simulink model "ex5_3_flowchart"  (R2018b)
settings: Solver=VariableStepAuto  StartTime=0.0  StopTime=20  RelTol=1e-3
settings Model: Creator=HYJ  LastModifiedBy=HYJ

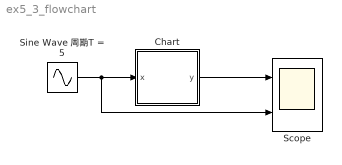
== system ex5_3_flowchart ==
  Chart : Stateflow chart  TreatAsAtomicUnit=on
  Scope : Scope  NumInputPorts=2
  Sine Wave 周期T = 5 : Sin  Frequency=0.2  SampleTime=0
  wires:
  Sine Wave 周期T = 5/1 -> Scope/2, Chart/1(x)
  Chart/1(y) -> Scope/1

== stateflow chart ex5_3_flowchart/Chart ==
  (default) -> (junction 7)
  (junction 7) -> (junction 9) [order 1] : [x>0.8]
  (junction 7) -> (junction 11) [order 2]
  (junction 9) -> (junction 12) : {y=0.3*x;}
  (junction 11) -> (junction 16) [order 1] : [x<=0.8 && x>=0.4]
  (junction 11) -> (junction 20) [order 2] : {y=x;}
  (junction 16) -> (junction 15) : {y=0.2*x;}
  (junction 15) -> (junction 20)
  (junction 12) -> (junction 15)
  (junction 20) -> (junction 23)
  data: x input; y output
